simulink model "eightbitadderdesign"  (R2014a)
settings: Solver=ode45  StartTime=0.0  StopTime=10.0  RelTol=1e-3
libraries: hdlsllib x17
settings Model: Creator=Andrew  LastModifiedBy=Andrew

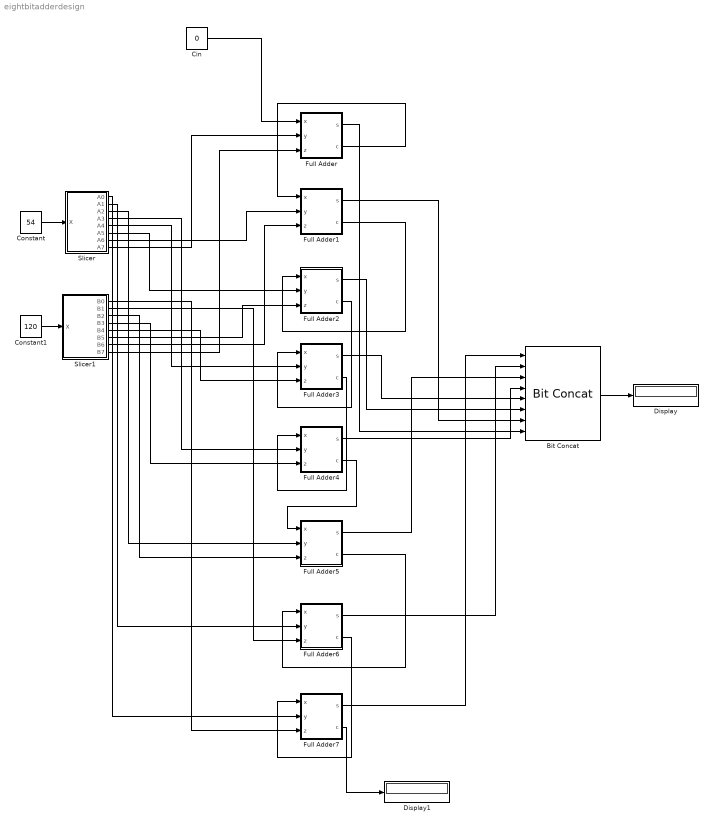
== system eightbitadderdesign ==
  Bit Concat : hdlsllib/HDL Operations/Bit Concat  numInputs=8
  Cin : Constant  Value=0  OutDataTypeStr=double
  Constant : Constant  Value=54  OutDataTypeStr=int8
  Constant1 : Constant  Value=120  OutDataTypeStr=int8
  Display : Display
  Display1 : Display
  Full Adder : Subsystem
  Full Adder1 : Subsystem
  Full Adder2 : Subsystem
  Full Adder3 : Subsystem
  Full Adder4 : Subsystem
  Full Adder5 : Subsystem
  Full Adder6 : Subsystem
  Full Adder7 : Subsystem
  Slicer : Subsystem
  Slicer1 : Subsystem
  wires:
  Cin/1 -> Full Adder/1(x)
  Full Adder/2(c) -> Full Adder1/1(x)
  Full Adder1/2(c) -> Full Adder2/1(x)
  Full Adder2/2(c) -> Full Adder3/1(x)
  Full Adder3/2(c) -> Full Adder4/1(x)
  Full Adder4/2(c) -> Full Adder5/1(x)
  Full Adder5/2(c) -> Full Adder6/1(x)
  Full Adder6/2(c) -> Full Adder7/1(x)
  Full Adder7/2(c) -> Display1/1
  Constant1/1 -> Slicer1/1(X)
  Constant/1 -> Slicer/1(X)
  Bit Concat/1 -> Display/1
  Slicer/8(A7) -> Full Adder/2(y)
  Slicer/7(A6) -> Full Adder1/2(y)
  Slicer/6(A5) -> Full Adder2/2(y)
  Slicer/5(A4) -> Full Adder3/2(y)
  Slicer/4(A3) -> Full Adder4/2(y)
  Slicer/3(A2) -> Full Adder5/2(y)
  Slicer/2(A1) -> Full Adder6/2(y)
  Slicer/1(A0) -> Full Adder7/2(y)
  Slicer1/8(B7) -> Full Adder/3(z)
  Slicer1/7(B6) -> Full Adder1/3(z)
  Slicer1/6(B5) -> Full Adder2/3(z)
  Slicer1/5(B4) -> Full Adder3/3(z)
  Slicer1/4(B3) -> Full Adder4/3(z)
  Slicer1/3(B2) -> Full Adder5/3(z)
  Slicer1/2(B1) -> Full Adder6/3(z)
  Slicer1/1(B0) -> Full Adder7/3(z)
  Full Adder7/1(s) -> Bit Concat/1
  Full Adder6/1(s) -> Bit Concat/2
  Full Adder5/1(s) -> Bit Concat/3
  Full Adder4/1(s) -> Bit Concat/4
  Full Adder3/1(s) -> Bit Concat/5
  Full Adder2/1(s) -> Bit Concat/6
  Full Adder1/1(s) -> Bit Concat/7
  Full Adder/1(s) -> Bit Concat/8

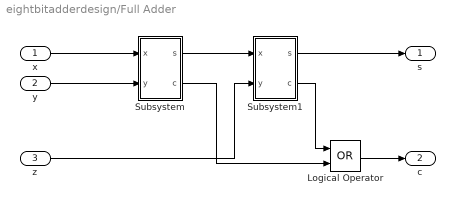
== system eightbitadderdesign/Full Adder ==
  x : Inport
  y : Inport  Port=2
  z : Inport  Port=3
  Logical Operator : Logic  Operator=OR  AllPortsSameDT=off  OutDataTypeStr=boolean
  Subsystem : Subsystem
  Subsystem1 : Subsystem
  s : Outport
  c : Outport  Port=2
  wires:
  Subsystem1/2(c) -> Logical Operator/1
  x/1 -> Subsystem/1(x)
  y/1 -> Subsystem/2(y)
  Subsystem/2(c) -> Logical Operator/2
  Subsystem/1(s) -> Subsystem1/1(x)
  z/1 -> Subsystem1/2(y)
  Subsystem1/1(s) -> s/1
  Logical Operator/1 -> c/1

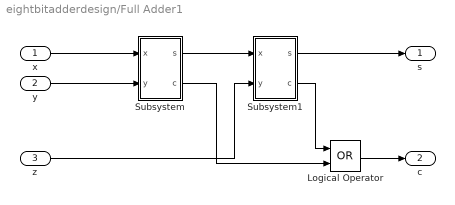
== system eightbitadderdesign/Full Adder1 ==
  x : Inport
  y : Inport  Port=2
  z : Inport  Port=3
  Logical Operator : Logic  Operator=OR  AllPortsSameDT=off  OutDataTypeStr=boolean
  Subsystem : Subsystem
  Subsystem1 : Subsystem
  s : Outport
  c : Outport  Port=2
  wires:
  Subsystem1/2(c) -> Logical Operator/1
  x/1 -> Subsystem/1(x)
  y/1 -> Subsystem/2(y)
  Subsystem/2(c) -> Logical Operator/2
  Subsystem/1(s) -> Subsystem1/1(x)
  z/1 -> Subsystem1/2(y)
  Subsystem1/1(s) -> s/1
  Logical Operator/1 -> c/1

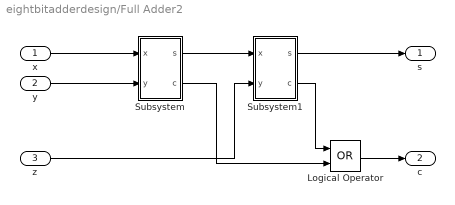
== system eightbitadderdesign/Full Adder2 ==
  x : Inport
  y : Inport  Port=2
  z : Inport  Port=3
  Logical Operator : Logic  Operator=OR  AllPortsSameDT=off  OutDataTypeStr=boolean
  Subsystem : Subsystem
  Subsystem1 : Subsystem
  s : Outport
  c : Outport  Port=2
  wires:
  Subsystem1/2(c) -> Logical Operator/1
  x/1 -> Subsystem/1(x)
  y/1 -> Subsystem/2(y)
  Subsystem/2(c) -> Logical Operator/2
  Subsystem/1(s) -> Subsystem1/1(x)
  z/1 -> Subsystem1/2(y)
  Subsystem1/1(s) -> s/1
  Logical Operator/1 -> c/1

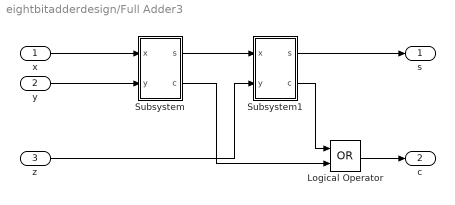
== system eightbitadderdesign/Full Adder3 ==
  x : Inport
  y : Inport  Port=2
  z : Inport  Port=3
  Logical Operator : Logic  Operator=OR  AllPortsSameDT=off  OutDataTypeStr=boolean
  Subsystem : Subsystem
  Subsystem1 : Subsystem
  s : Outport
  c : Outport  Port=2
  wires:
  Subsystem1/2(c) -> Logical Operator/1
  x/1 -> Subsystem/1(x)
  y/1 -> Subsystem/2(y)
  Subsystem/2(c) -> Logical Operator/2
  Subsystem/1(s) -> Subsystem1/1(x)
  z/1 -> Subsystem1/2(y)
  Subsystem1/1(s) -> s/1
  Logical Operator/1 -> c/1

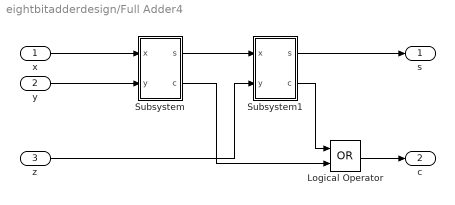
== system eightbitadderdesign/Full Adder4 ==
  x : Inport
  y : Inport  Port=2
  z : Inport  Port=3
  Logical Operator : Logic  Operator=OR  AllPortsSameDT=off  OutDataTypeStr=boolean
  Subsystem : Subsystem
  Subsystem1 : Subsystem
  s : Outport
  c : Outport  Port=2
  wires:
  Subsystem1/2(c) -> Logical Operator/1
  x/1 -> Subsystem/1(x)
  y/1 -> Subsystem/2(y)
  Subsystem/2(c) -> Logical Operator/2
  Subsystem/1(s) -> Subsystem1/1(x)
  z/1 -> Subsystem1/2(y)
  Subsystem1/1(s) -> s/1
  Logical Operator/1 -> c/1

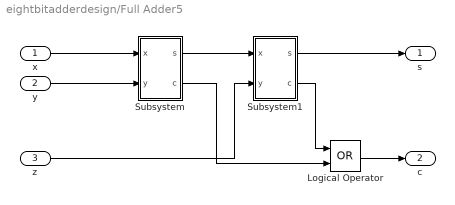
== system eightbitadderdesign/Full Adder5 ==
  x : Inport
  y : Inport  Port=2
  z : Inport  Port=3
  Logical Operator : Logic  Operator=OR  AllPortsSameDT=off  OutDataTypeStr=boolean
  Subsystem : Subsystem
  Subsystem1 : Subsystem
  s : Outport
  c : Outport  Port=2
  wires:
  Subsystem1/2(c) -> Logical Operator/1
  x/1 -> Subsystem/1(x)
  y/1 -> Subsystem/2(y)
  Subsystem/2(c) -> Logical Operator/2
  Subsystem/1(s) -> Subsystem1/1(x)
  z/1 -> Subsystem1/2(y)
  Subsystem1/1(s) -> s/1
  Logical Operator/1 -> c/1

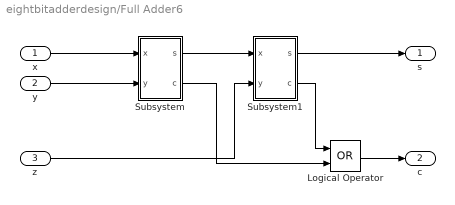
== system eightbitadderdesign/Full Adder6 ==
  x : Inport
  y : Inport  Port=2
  z : Inport  Port=3
  Logical Operator : Logic  Operator=OR  AllPortsSameDT=off  OutDataTypeStr=boolean
  Subsystem : Subsystem
  Subsystem1 : Subsystem
  s : Outport
  c : Outport  Port=2
  wires:
  Subsystem1/2(c) -> Logical Operator/1
  x/1 -> Subsystem/1(x)
  y/1 -> Subsystem/2(y)
  Subsystem/2(c) -> Logical Operator/2
  Subsystem/1(s) -> Subsystem1/1(x)
  z/1 -> Subsystem1/2(y)
  Subsystem1/1(s) -> s/1
  Logical Operator/1 -> c/1

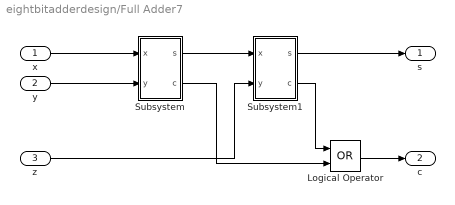
== system eightbitadderdesign/Full Adder7 ==
  x : Inport
  y : Inport  Port=2
  z : Inport  Port=3
  Logical Operator : Logic  Operator=OR  AllPortsSameDT=off  OutDataTypeStr=boolean
  Subsystem : Subsystem
  Subsystem1 : Subsystem
  s : Outport
  c : Outport  Port=2
  wires:
  Subsystem1/2(c) -> Logical Operator/1
  x/1 -> Subsystem/1(x)
  y/1 -> Subsystem/2(y)
  Subsystem/2(c) -> Logical Operator/2
  Subsystem/1(s) -> Subsystem1/1(x)
  z/1 -> Subsystem1/2(y)
  Subsystem1/1(s) -> s/1
  Logical Operator/1 -> c/1

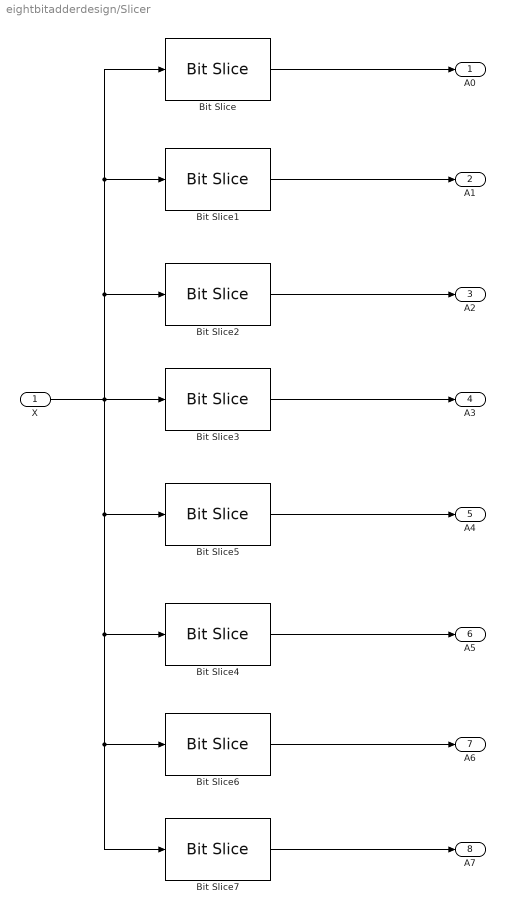
== system eightbitadderdesign/Slicer ==
  X : Inport  OutDataTypeStr=int8  SampleTime=1
  Bit Slice : hdlsllib/HDL Operations/Bit Slice  lidx=7  ridx=7
  Bit Slice1 : hdlsllib/HDL Operations/Bit Slice  lidx=6  ridx=6
  Bit Slice2 : hdlsllib/HDL Operations/Bit Slice  lidx=5  ridx=5
  Bit Slice3 : hdlsllib/HDL Operations/Bit Slice  lidx=4  ridx=4
  Bit Slice4 : hdlsllib/HDL Operations/Bit Slice  lidx=2  ridx=2
  Bit Slice5 : hdlsllib/HDL Operations/Bit Slice  lidx=3  ridx=3
  Bit Slice6 : hdlsllib/HDL Operations/Bit Slice  lidx=1  ridx=1
  Bit Slice7 : hdlsllib/HDL Operations/Bit Slice  lidx=0  ridx=0
  A0 : Outport
  A1 : Outport  Port=2
  A2 : Outport  Port=3
  A3 : Outport  Port=4
  A4 : Outport  Port=5
  A5 : Outport  Port=6
  A6 : Outport  Port=7
  A7 : Outport  Port=8
  wires:
  X/1 -> Bit Slice7/1, Bit Slice6/1, Bit Slice4/1, Bit Slice5/1, Bit Slice/1, Bit Slice1/1, Bit Slice2/1, Bit Slice3/1
  Bit Slice/1 -> A0/1
  Bit Slice7/1 -> A7/1
  Bit Slice3/1 -> A3/1
  Bit Slice1/1 -> A1/1
  Bit Slice5/1 -> A4/1
  Bit Slice2/1 -> A2/1
  Bit Slice4/1 -> A5/1
  Bit Slice6/1 -> A6/1

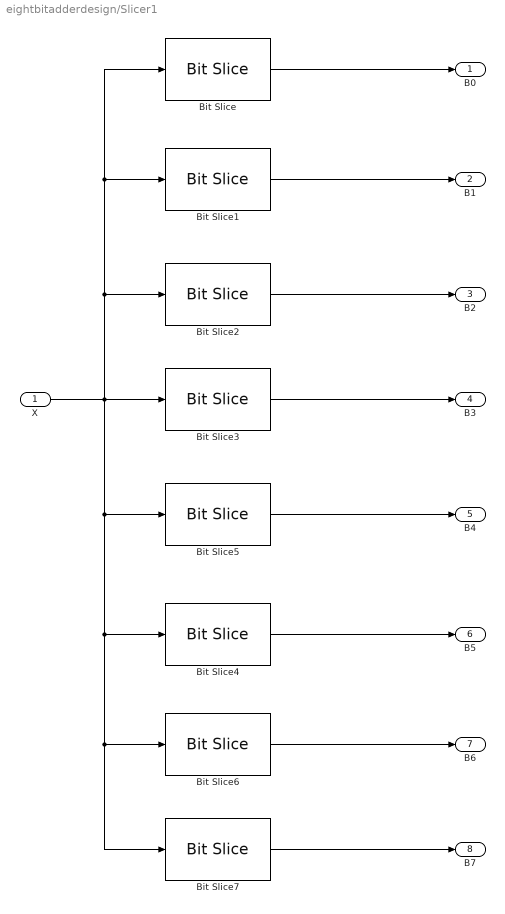
== system eightbitadderdesign/Slicer1 ==
  X : Inport  OutDataTypeStr=int8  SampleTime=1
  Bit Slice : hdlsllib/HDL Operations/Bit Slice  lidx=7  ridx=7
  Bit Slice1 : hdlsllib/HDL Operations/Bit Slice  lidx=6  ridx=6
  Bit Slice2 : hdlsllib/HDL Operations/Bit Slice  lidx=5  ridx=5
  Bit Slice3 : hdlsllib/HDL Operations/Bit Slice  lidx=4  ridx=4
  Bit Slice4 : hdlsllib/HDL Operations/Bit Slice  lidx=2  ridx=2
  Bit Slice5 : hdlsllib/HDL Operations/Bit Slice  lidx=3  ridx=3
  Bit Slice6 : hdlsllib/HDL Operations/Bit Slice  lidx=1  ridx=1
  Bit Slice7 : hdlsllib/HDL Operations/Bit Slice  lidx=0  ridx=0
  B0 : Outport
  B1 : Outport  Port=2
  B2 : Outport  Port=3
  B3 : Outport  Port=4
  B4 : Outport  Port=5
  B5 : Outport  Port=6
  B6 : Outport  Port=7
  B7 : Outport  Port=8
  wires:
  X/1 -> Bit Slice7/1, Bit Slice6/1, Bit Slice4/1, Bit Slice5/1, Bit Slice/1, Bit Slice1/1, Bit Slice2/1, Bit Slice3/1
  Bit Slice/1 -> B0/1
  Bit Slice7/1 -> B7/1
  Bit Slice3/1 -> B3/1
  Bit Slice1/1 -> B1/1
  Bit Slice5/1 -> B4/1
  Bit Slice2/1 -> B2/1
  Bit Slice4/1 -> B5/1
  Bit Slice6/1 -> B6/1

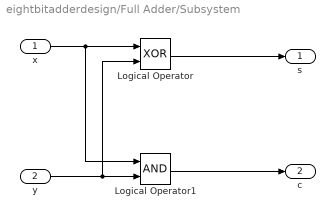
== system eightbitadderdesign/Full Adder/Subsystem ==
  x : Inport
  y : Inport  Port=2
  Logical Operator : Logic  Operator=XOR  AllPortsSameDT=off  OutDataTypeStr=boolean
  Logical Operator1 : Logic  AllPortsSameDT=off  OutDataTypeStr=boolean
  s : Outport
  c : Outport  Port=2
  wires:
  x/1 -> Logical Operator1/1, Logical Operator/1
  Logical Operator1/1 -> c/1
  y/1 -> Logical Operator/2, Logical Operator1/2
  Logical Operator/1 -> s/1

== system eightbitadderdesign/Full Adder/Subsystem1 ==
  x : Inport
  y : Inport  Port=2
  Logical Operator : Logic  Operator=XOR  AllPortsSameDT=off  OutDataTypeStr=boolean
  Logical Operator1 : Logic  AllPortsSameDT=off  OutDataTypeStr=boolean
  s : Outport
  c : Outport  Port=2
  wires:
  x/1 -> Logical Operator1/1, Logical Operator/1
  Logical Operator1/1 -> c/1
  y/1 -> Logical Operator/2, Logical Operator1/2
  Logical Operator/1 -> s/1

== system eightbitadderdesign/Full Adder1/Subsystem ==
  x : Inport
  y : Inport  Port=2
  Logical Operator : Logic  Operator=XOR  AllPortsSameDT=off  OutDataTypeStr=boolean
  Logical Operator1 : Logic  AllPortsSameDT=off  OutDataTypeStr=boolean
  s : Outport
  c : Outport  Port=2
  wires:
  x/1 -> Logical Operator1/1, Logical Operator/1
  Logical Operator1/1 -> c/1
  y/1 -> Logical Operator/2, Logical Operator1/2
  Logical Operator/1 -> s/1

== system eightbitadderdesign/Full Adder1/Subsystem1 ==
  x : Inport
  y : Inport  Port=2
  Logical Operator : Logic  Operator=XOR  AllPortsSameDT=off  OutDataTypeStr=boolean
  Logical Operator1 : Logic  AllPortsSameDT=off  OutDataTypeStr=boolean
  s : Outport
  c : Outport  Port=2
  wires:
  x/1 -> Logical Operator1/1, Logical Operator/1
  Logical Operator1/1 -> c/1
  y/1 -> Logical Operator/2, Logical Operator1/2
  Logical Operator/1 -> s/1

== system eightbitadderdesign/Full Adder2/Subsystem ==
  x : Inport
  y : Inport  Port=2
  Logical Operator : Logic  Operator=XOR  AllPortsSameDT=off  OutDataTypeStr=boolean
  Logical Operator1 : Logic  AllPortsSameDT=off  OutDataTypeStr=boolean
  s : Outport
  c : Outport  Port=2
  wires:
  x/1 -> Logical Operator1/1, Logical Operator/1
  Logical Operator1/1 -> c/1
  y/1 -> Logical Operator/2, Logical Operator1/2
  Logical Operator/1 -> s/1

== system eightbitadderdesign/Full Adder2/Subsystem1 ==
  x : Inport
  y : Inport  Port=2
  Logical Operator : Logic  Operator=XOR  AllPortsSameDT=off  OutDataTypeStr=boolean
  Logical Operator1 : Logic  AllPortsSameDT=off  OutDataTypeStr=boolean
  s : Outport
  c : Outport  Port=2
  wires:
  x/1 -> Logical Operator1/1, Logical Operator/1
  Logical Operator1/1 -> c/1
  y/1 -> Logical Operator/2, Logical Operator1/2
  Logical Operator/1 -> s/1

== system eightbitadderdesign/Full Adder3/Subsystem ==
  x : Inport
  y : Inport  Port=2
  Logical Operator : Logic  Operator=XOR  AllPortsSameDT=off  OutDataTypeStr=boolean
  Logical Operator1 : Logic  AllPortsSameDT=off  OutDataTypeStr=boolean
  s : Outport
  c : Outport  Port=2
  wires:
  x/1 -> Logical Operator1/1, Logical Operator/1
  Logical Operator1/1 -> c/1
  y/1 -> Logical Operator/2, Logical Operator1/2
  Logical Operator/1 -> s/1

== system eightbitadderdesign/Full Adder3/Subsystem1 ==
  x : Inport
  y : Inport  Port=2
  Logical Operator : Logic  Operator=XOR  AllPortsSameDT=off  OutDataTypeStr=boolean
  Logical Operator1 : Logic  AllPortsSameDT=off  OutDataTypeStr=boolean
  s : Outport
  c : Outport  Port=2
  wires:
  x/1 -> Logical Operator1/1, Logical Operator/1
  Logical Operator1/1 -> c/1
  y/1 -> Logical Operator/2, Logical Operator1/2
  Logical Operator/1 -> s/1

== system eightbitadderdesign/Full Adder4/Subsystem ==
  x : Inport
  y : Inport  Port=2
  Logical Operator : Logic  Operator=XOR  AllPortsSameDT=off  OutDataTypeStr=boolean
  Logical Operator1 : Logic  AllPortsSameDT=off  OutDataTypeStr=boolean
  s : Outport
  c : Outport  Port=2
  wires:
  x/1 -> Logical Operator1/1, Logical Operator/1
  Logical Operator1/1 -> c/1
  y/1 -> Logical Operator/2, Logical Operator1/2
  Logical Operator/1 -> s/1

== system eightbitadderdesign/Full Adder4/Subsystem1 ==
  x : Inport
  y : Inport  Port=2
  Logical Operator : Logic  Operator=XOR  AllPortsSameDT=off  OutDataTypeStr=boolean
  Logical Operator1 : Logic  AllPortsSameDT=off  OutDataTypeStr=boolean
  s : Outport
  c : Outport  Port=2
  wires:
  x/1 -> Logical Operator1/1, Logical Operator/1
  Logical Operator1/1 -> c/1
  y/1 -> Logical Operator/2, Logical Operator1/2
  Logical Operator/1 -> s/1

== system eightbitadderdesign/Full Adder5/Subsystem ==
  x : Inport
  y : Inport  Port=2
  Logical Operator : Logic  Operator=XOR  AllPortsSameDT=off  OutDataTypeStr=boolean
  Logical Operator1 : Logic  AllPortsSameDT=off  OutDataTypeStr=boolean
  s : Outport
  c : Outport  Port=2
  wires:
  x/1 -> Logical Operator1/1, Logical Operator/1
  Logical Operator1/1 -> c/1
  y/1 -> Logical Operator/2, Logical Operator1/2
  Logical Operator/1 -> s/1

== system eightbitadderdesign/Full Adder5/Subsystem1 ==
  x : Inport
  y : Inport  Port=2
  Logical Operator : Logic  Operator=XOR  AllPortsSameDT=off  OutDataTypeStr=boolean
  Logical Operator1 : Logic  AllPortsSameDT=off  OutDataTypeStr=boolean
  s : Outport
  c : Outport  Port=2
  wires:
  x/1 -> Logical Operator1/1, Logical Operator/1
  Logical Operator1/1 -> c/1
  y/1 -> Logical Operator/2, Logical Operator1/2
  Logical Operator/1 -> s/1

== system eightbitadderdesign/Full Adder6/Subsystem ==
  x : Inport
  y : Inport  Port=2
  Logical Operator : Logic  Operator=XOR  AllPortsSameDT=off  OutDataTypeStr=boolean
  Logical Operator1 : Logic  AllPortsSameDT=off  OutDataTypeStr=boolean
  s : Outport
  c : Outport  Port=2
  wires:
  x/1 -> Logical Operator1/1, Logical Operator/1
  Logical Operator1/1 -> c/1
  y/1 -> Logical Operator/2, Logical Operator1/2
  Logical Operator/1 -> s/1

== system eightbitadderdesign/Full Adder6/Subsystem1 ==
  x : Inport
  y : Inport  Port=2
  Logical Operator : Logic  Operator=XOR  AllPortsSameDT=off  OutDataTypeStr=boolean
  Logical Operator1 : Logic  AllPortsSameDT=off  OutDataTypeStr=boolean
  s : Outport
  c : Outport  Port=2
  wires:
  x/1 -> Logical Operator1/1, Logical Operator/1
  Logical Operator1/1 -> c/1
  y/1 -> Logical Operator/2, Logical Operator1/2
  Logical Operator/1 -> s/1

== system eightbitadderdesign/Full Adder7/Subsystem ==
  x : Inport
  y : Inport  Port=2
  Logical Operator : Logic  Operator=XOR  AllPortsSameDT=off  OutDataTypeStr=boolean
  Logical Operator1 : Logic  AllPortsSameDT=off  OutDataTypeStr=boolean
  s : Outport
  c : Outport  Port=2
  wires:
  x/1 -> Logical Operator1/1, Logical Operator/1
  Logical Operator1/1 -> c/1
  y/1 -> Logical Operator/2, Logical Operator1/2
  Logical Operator/1 -> s/1

== system eightbitadderdesign/Full Adder7/Subsystem1 ==
  x : Inport
  y : Inport  Port=2
  Logical Operator : Logic  Operator=XOR  AllPortsSameDT=off  OutDataTypeStr=boolean
  Logical Operator1 : Logic  AllPortsSameDT=off  OutDataTypeStr=boolean
  s : Outport
  c : Outport  Port=2
  wires:
  x/1 -> Logical Operator1/1, Logical Operator/1
  Logical Operator1/1 -> c/1
  y/1 -> Logical Operator/2, Logical Operator1/2
  Logical Operator/1 -> s/1
